simulink model "gravityGradient_test"  (R2018b)
settings: Solver=VariableStepAuto  StartTime=0.0  StopTime=0  RelTol=1e-3
values from neighbouring files (symbols this model uses):
  state = [qd;reci;w0;v]    [gravityGradient_test_init.m]
libraries: gravityGrad_Lib x1
settings Model: Creator=devantormey  LastModifiedBy=IvanMachuca

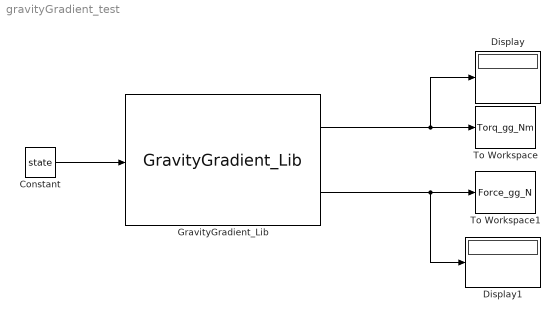
== system gravityGradient_test ==
  Constant : Constant  Value=state
  Display : Display
  Display1 : Display
  "GravityGradient_Lib " : gravityGrad_Lib/GravityGradient_Lib   SystemSampleTime=-1
  To Workspace : ToWorkspace  VariableName=Torq_gg_Nm  SampleTime=-1
      settings: Save2DSignal=2-D array (concatenate along first dimension)
  To Workspace1 : ToWorkspace  VariableName=Force_gg_N  SampleTime=-1
      settings: Save2DSignal=2-D array (concatenate along first dimension)
  wires:
  "GravityGradient_Lib "/2 -> To Workspace1/1, Display1/1
  "GravityGradient_Lib "/1 -> To Workspace/1, Display/1
  Constant/1 -> "GravityGradient_Lib "/1
